simulink model "OnBoardMatlabExpo3"  (R2015b)
settings: Solver=FixedStepDiscrete  SolverMode=SingleTasking  StartTime=0.0  StopTime=10.0  FixedStep=0.002  RelTol=1e-3
PreLoadFcn:
  | waijung.modelPreload; % Required for working with Waijung Blockset. Do not remove.
undefined symbols (not defined in the file): CPHA_1Edge, CPOL_Low, Duplex, FirstBit_MSB, Full, Link, LQFP100, ST, STM32F407VG, STM32F4DISCOVERY
libraries: simulink x12, stm32f4_io_lib x7, cube_lib x3, stm32f4_spi_lib x3, stm32f4_device_config_lib x1, BC_USB x1, stm32f4_adc_lib x1
(part 1 of 2)
CloseFcn:
  | waijung.modelClose; % Required for working with Waijung Blockset. Do not remove.
settings Model: Creator=Hi  LastModifiedBy=Stefan
settings DataIOCC: SaveFormat=Array
settings OptimizationCC: OptimizeModelRefInitCode=on  LifeSpan=1
settings HardwareCC: ProdBitPerPointer=32  ProdLargestAtomicFloat=None  ProdIntDivRoundTo=Undefined  ProdWordSize=32  ProdHWDeviceType=ARM Compatible->Cortex - M4  TargetEndianess=LittleEndian  TargetHWDeviceType=ARM Compatible->Cortex - M4
settings RTWCC: SystemTargetFile=stm32f4.tlc  GenerateMakefile=off  TemplateMakefile=ert_default_tmf  Description=STM32F4 Target
settings CodeAppCC: ForceParamTrailComments=on  IgnoreCustomStorageClasses=off  OperatorAnnotations=on  SimulinkDataObjDesc=on  InsertBlockDesc=on  MATLABSourceComments=on
settings STFCustomTargetCC: ModelReferenceCompliant=off  ConcurrentExecutionCompliant=off  GeneratePreprocessorConditionals=Use local settings  CombineOutputUpdateFcns=on  ERTCustomFileBanners=on  SupportContinuousTime=off  SupportNonInlinedSFcns=off  MATLABClassNameForMDSCustomization=Simulink.SoftwareTarget.ERTCustomization  CPPClassGenCompliant=off  GRTInterface=off  SystemTargetFile=stm32f4.tlc
settings ERTTargetCC: ModelReferenceCompliant=off  ParMdlRefBuildCompliant=off  CompOptLevelCompliant=off  ConcurrentExecutionCompliant=off  ERTFirstTimeCompliant=off  ModelStepFunctionPrototypeControlCompliant=off  CPPClassGenCompliant=off  UseToolchainInfoCompliant=off  ERTSrcFileBannerTemplate=stm32f4_code_template.cgt  ERTHdrFileBannerTemplate=stm32f4_code_template.cgt  ERTDataSrcFileTemplate=stm32f4_code_template.cgt  ERTDataHdrFileTemplate=stm32f4_code_template.cgt  ERTCustomFileTemplate=stm32f4_file_process.tlc
settings ConfigComp: CovModelRefEnable=Off

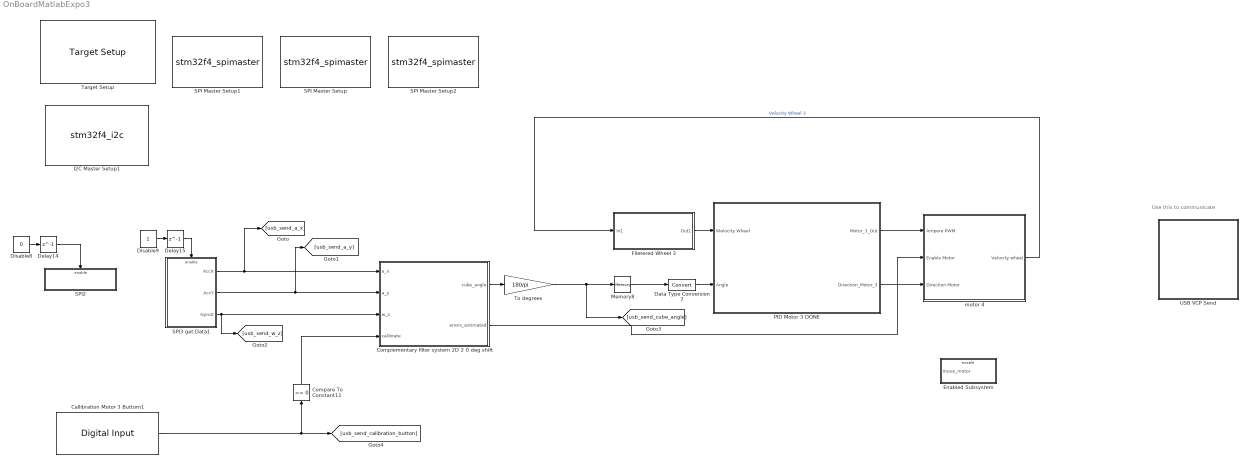
== system OnBoardMatlabExpo3 ==
  note: Use this to communicate
  Callibration Motor 3 Buttom1 : stm32f4_io_lib/Digital Input  port=E  speed=100  porttype=Pull Up  porttypestr=UP  use_pin0=off  use_pin1=off  use_pin2=off  use_pin3=off  use_pin4=off  use_pin5=off  use_pin6=off  use_pin7=off  use_pin8=off  use_pin9=off  use_pin10=on  use_pin11=off  use_pin12=off  use_pin13=off  use_pin14=off  use_pin15=off  pinstr=GPIO_Pin_10  usedpinarray="[0  0  0  0  0  0  0  0  0  0  1  0  0  0  0  0]"  bitbandingstr="#define CallibrationMotor3Buttom1_E10 Peripheral_BB(GPIOE->IDR, 10)  /* Output pin */"  sampletime=0.002  sampletimestr=0.002  blockid=CallibrationMotor3Buttom1  enablecustomportlabel=off  glabalinit=off  cinputportlabel=In1, In2  coutputportlabel=Out1, Out2
  Compare To Constant11 : simulink/Logic and Bit Operations/Compare To Constant  relop===  const=0  OutDataTypeStr=boolean  ZeroCross=off
  Complementary filter system 2D 2 0 deg shift : Subsystem  AncestorBlock=cube_lib/Complementary filter system 2D 2 0 deg shift
  Data Type Conversion7 : DataTypeConversion
  Delay14 : Delay  DelayLength=1  InitialCondition=1
  Delay15 : Delay  DelayLength=1  InitialCondition=0
  Disable8 : Constant  Value=0
  Disable9 : Constant
  Enabled Subsystem : Subsystem  TreatAsAtomicUnit=on
  Filetered Wheel 3 : Subsystem
  I2C Master Setup1 : S-Function  FunctionName=stm32f4_i2c  Parameters=configuration,module,transfer,clkspeed,timeout,sdapin,sclpin,writecount,readcount,inputtypearray,outputtypearray,confstr,sampletime,sampletimestr,blockid  SFunctionDeploymentMode=off  EnableBusSupport=off  mask(stm32f4_i2c){configuration=Setup, module=1, lastmodule=1, transfer=Blocking, dutycycle=TLow/THigh = 2, clkspeed=400, timeout=25, writecount=0, readcount=0, sdapin=B7, sclpin=B6, waitwritetime=0, inputtypearray=[0], outputtypearray=[0], confstr=["B","7","B","6","1","1","6","0","I2C_DutyCycle_2","0","off"], sampletime=-1, sampletimestr=0.002, blockid=I2CMasterSetup1}
      mask prompts: module "I2C Module"; lastmodule "Last module"; transfer "Transfer mode"; dutycycle "Duty cycle in fast mode"; clkspeed "Clock speed (kHz)"; timeout "Timeout (ms)"; writecount "Bytes write count"; readcount "Bytes read count"; sdapin "SDA pin"; sclpin "SCL pin"; waitwritetime "Wait write time (ms), default is 0"; inputtypearray "Input type array"; outputtypearray "Output type array"; confstr "Configuration string"; sampletime "Sample time (sec)"; sampletimestr "Compiled sample time (sec) in string"
      mask init:
      | stm32f4_i2c_callback('init');
      mask Help: web(fullfile(waijungdocroot,'stm32f4_i2c_setup.htm'), '-browser')
      mask TypeOptions configuration: Setup | Transaction
      mask Callback configuration: stm32f4_i2c_callback('configuration');
      mask TypeOptions module: 1 | 2 | 3
      mask Callback module: stm32f4_i2c_callback('module');
      mask TypeOptions transfer: Blocking | Non-blocking
      mask TypeOptions dutycycle: TLow/THigh = 16/9 | TLow/THigh = 2
      mask Callback dutycycle: stm32f4_i2c_callback('dutycycle');
      mask Callback writecount: stm32f4_i2c_callback('writecount');
      mask Callback readcount: stm32f4_i2c_callback('readcount');
      mask TypeOptions sdapin: - | B7 | B9
      mask Callback sdapin: stm32f4_i2c_callback('sdapin');
      mask TypeOptions sclpin: - | B6 | B8
      mask Callback sclpin: stm32f4_i2c_callback('sclpin');
      mask Callback confstr: stm32f4_i2c_callback('confstr');
      mask Callback sampletime: stm32f4_i2c_callback('sampletime');
      mask Callback sampletimestr: stm32f4_i2c_callback('sampletimestr');
      mask Callback blockid: stm32f4_i2c_callback('blockid');
      mask Display: text(0.5, 0.5, 'Module: I2C1\nClock: 400kHz\nSDA/SCL Pin: B7/B6','ver','middle','hor','center');
  Memory8 : Memory  InheritSampleTime=on
  "PID Motor 3 DONE " : Subsystem
  SPI Master Setup : S-Function  FunctionName=stm32f4_spimaster  Parameters=mode,configuration,module,datacount,inputtypearray,outputtypearray,confstr,sampletime,sampletimestr,blockid  SFunctionDeploymentMode=off  EnableBusSupport=off  mask(stm32f4_spimaster){configuration=Setup, module=2, mode=Write, lastmodule=2, direction=Full-Duplex, dataformat=8bit/ FirstBit_MSB, prescaler=32, lastpclk=42000000, baudrate=1312500, cpolcpha=CPOL_Low/ CPHA_1Edge, datacount=0, nssmode=Software, nsspin=Not used, softnssport=B, softnsspin=12, sckpin=B13, misopin=B14, mosipin=B15, pintype=Push Pull, pulltype=Pull Up, nssdelay=0, inputtypearray=[0], outputtypearray=[0], confstr=["SPI_Direction_2Lines_FullDuplex","8b","MSB","Low","1Edge","32","Soft","0","x","x","1","B","12","1","B","13","1","B","14","1","B","15","0","1","0","0","0","0","0","0","0","PP","0","UP"], sampletime=-1, sampletimestr=0.002, blockid=SPIMasterSetup}
      mask prompts: module "SPI Module:"; lastmodule "Last module:"; dataformat "Data format:"; prescaler "Buad rate prescaler: Pclk/"; lastpclk "Last PCLK"; baudrate "Baud rate (Hz)"; cpolcpha "Clock polarity (CPOL)/ Clock phase (CPHA):"; datacount "Data Write count:"; nssmode "Slave/chip select (nSS, nCS) mode"; nsspin "Slave/chip select (nSS, nCS) pin"; softnssport "Slave/chip select port (nSS, nCS)"; softnsspin "Slave/chip select pin (nSS, nCS)"; sckpin "SCLK pin:"; misopin "MISO pin:"; mosipin "MOSI pin:"; pintype "Pin type (Push-Pull/Open-Drain)"; pulltype "Pull Type (Up/Down)"; nssdelay "Data delay time, uS:"; inputtypearray "Input type array"; outputtypearray "Output type array"; confstr "Configuration string"; sampletime "Sample time (sec)"; sampletimestr "Compiled sample time (sec) in string"
      mask help:
      | Direction:
      |  - Full-Duplex, use this mode when need to send and receive data at same clock.
      |  - Half-Duplex_Tx, this mode is to transmit data to slave only. Pin MISO (Rx) can be free for other function.
      |  - Half-Duplex_Rx, this mode is to receive data from slave only. Pin MOSIO (Tx) can be free for other function.
      | Data format:
      |   This configuration is depending on the specification of slave device.
      | Baud rate prescaler:
      |  - Use this prescaler to devide from the PCLK for SPI clock.
      |  - This Prescaler value is auto determine corresponding to baudrate setting and selected SPI module.
      | Baud rate (Hz):
      |  - Select baud rate for SPI clock. Please check the maximum clock support for target slave device.
      | Clock polarity and Clock phase:
      |  - This configuration parameter is depending on slave device.
      |  - See waijung help for more description.
      | Slave/chip select mode:
      |  - Hardware, use hardware SPI module for slave select (or chip select) pin.
      |  - Software, this mode allow any available pin for slave select (or chip select) function.
      |  - Custom, SPI block did not control slave select pin. User may use Digital Output block to control by costom.
      mask init:
      | stm32f4_spimaster_callback('init');
      mask Help: web(fullfile(waijungdocroot,'stm32f4_spimaster_setup.htm'), '-browser')
      mask TypeOptions configuration: Setup | Transaction
      mask Callback configuration: stm32f4_spimaster_callback('configuration');
      mask TypeOptions module: 1 | 2 | 3
      mask Callback module: stm32f4_spimaster_callback('module');
      mask TypeOptions mode: Read/ Write | Read | Write
      mask Callback mode: stm32f4_spimaster_callback('mode');
      mask TypeOptions direction: Full-Duplex | Half-Duplex_Tx | Half-Duplex_Rx
      mask Callback direction: stm32f4_spimaster_callback('direction');
      mask TypeOptions dataformat: 8bit/ FirstBit_MSB | 8bit/ FirstBit_LSB | 16bit/ FirstBit_MSB | 16bit/ FirstBit_LSB
      mask TypeOptions prescaler: 2 | 4 | 8 | 16 | 32 | 64 | 128 | 256
      mask TypeOptions baudrate: Not set | 21000000 | 10500000 | 5250000 | 2625000 | 1312500 | 656250 | 328125 | 164063
      mask Callback baudrate: stm32f4_spimaster_callback('baudrate');
      mask TypeOptions cpolcpha: CPOL_Low/ CPHA_1Edge | CPOL_Low/ CPHA_2Edge | CPOL_High/ CPHA_1Edge | CPOL_High/ CPHA_2Edge
      mask Callback datacount: stm32f4_spimaster_callback('datacount');
      mask TypeOptions nssmode: Hardware | Software | Custom
      mask Callback nssmode: stm32f4_spimaster_callback('nssmode');
      mask TypeOptions nsspin: Not used | B9 | B12
      mask TypeOptions softnssport: A | B | C | D | E | F | G | H | I
      mask TypeOptions softnsspin: 0 | 1 | 2 | 3 | 4 | 5 | 6 | 7 | 8 | 9 | 10 | 11 | 12 | 13 | 14 | 15
      mask TypeOptions sckpin: Not used | B10 | B13
      mask TypeOptions misopin: Not used | B14 | C2
      mask TypeOptions mosipin: Not used | B15 | C3
      mask TypeOptions pintype: Push Pull | Open Drain
      mask TypeOptions pulltype: None | Pull Up | Pull Down
      mask Callback confstr: stm32f4_spimaster_callback('confstr');
      mask Callback sampletime: stm32f4_spimaster_callback('sampletime');
      mask Callback sampletimestr: stm32f4_spimaster_callback('sampletimestr');
      mask Callback blockid: stm32f4_spimaster_callback('blockid');
      mask Display: text(0.5, 0.5, 'Module: SPI2 (Master)\nFull-Duplex\nBaudrate: 1312500','ver','middle','hor','center');
  SPI Master Setup1 : S-Function  FunctionName=stm32f4_spimaster  Parameters=mode,configuration,module,datacount,inputtypearray,outputtypearray,confstr,sampletime,sampletimestr,blockid  SFunctionDeploymentMode=off  EnableBusSupport=off  mask(stm32f4_spimaster){configuration=Setup, module=1, mode=Write, lastmodule=1, direction=Full-Duplex, dataformat=8bit/ FirstBit_MSB, prescaler=64, lastpclk=84000000, baudrate=1312500, cpolcpha=CPOL_Low/ CPHA_1Edge, datacount=0, nssmode=Software, nsspin=Not used, softnssport=C, softnsspin=5, sckpin=A5, misopin=A6, mosipin=A7, pintype=Push Pull, pulltype=Pull Up, nssdelay=0, inputtypearray=[0], outputtypearray=[0], confstr=["SPI_Direction_2Lines_FullDuplex","8b","MSB","Low","1Edge","64","Soft","0","x","x","1","C","5","1","A","5","1","A","6","1","A","7","1","0","1","0","0","0","0","0","0","PP","0","UP"], sampletime=-1, sampletimestr=0.002, blockid=SPIMasterSetup1}
      mask prompts: module "SPI Module:"; lastmodule "Last module:"; dataformat "Data format:"; prescaler "Buad rate prescaler: Pclk/"; lastpclk "Last PCLK"; baudrate "Baud rate (Hz)"; cpolcpha "Clock polarity (CPOL)/ Clock phase (CPHA):"; datacount "Data Write count:"; nssmode "Slave/chip select (nSS, nCS) mode"; nsspin "Slave/chip select (nSS, nCS) pin"; softnssport "Slave/chip select port (nSS, nCS)"; softnsspin "Slave/chip select pin (nSS, nCS)"; sckpin "SCLK pin:"; misopin "MISO pin:"; mosipin "MOSI pin:"; pintype "Pin type (Push-Pull/Open-Drain)"; pulltype "Pull Type (Up/Down)"; nssdelay "Data delay time, uS:"; inputtypearray "Input type array"; outputtypearray "Output type array"; confstr "Configuration string"; sampletime "Sample time (sec)"; sampletimestr "Compiled sample time (sec) in string"
      mask help:
      | Direction:
      |  - Full-Duplex, use this mode when need to send and receive data at same clock.
      |  - Half-Duplex_Tx, this mode is to transmit data to slave only. Pin MISO (Rx) can be free for other function.
      |  - Half-Duplex_Rx, this mode is to receive data from slave only. Pin MOSIO (Tx) can be free for other function.
      | Data format:
      |   This configuration is depending on the specification of slave device.
      | Baud rate prescaler:
      |  - Use this prescaler to devide from the PCLK for SPI clock.
      |  - This Prescaler value is auto determine corresponding to baudrate setting and selected SPI module.
      | Baud rate (Hz):
      |  - Select baud rate for SPI clock. Please check the maximum clock support for target slave device.
      | Clock polarity and Clock phase:
      |  - This configuration parameter is depending on slave device.
      |  - See waijung help for more description.
      | Slave/chip select mode:
      |  - Hardware, use hardware SPI module for slave select (or chip select) pin.
      |  - Software, this mode allow any available pin for slave select (or chip select) function.
      |  - Custom, SPI block did not control slave select pin. User may use Digital Output block to control by costom.
      mask init:
      | stm32f4_spimaster_callback('init');
      mask Help: web(fullfile(waijungdocroot,'stm32f4_spimaster_setup.htm'), '-browser')
      mask TypeOptions configuration: Setup | Transaction
      mask Callback configuration: stm32f4_spimaster_callback('configuration');
      mask TypeOptions module: 1 | 2 | 3
      mask Callback module: stm32f4_spimaster_callback('module');
      mask TypeOptions mode: Read/ Write | Read | Write
      mask Callback mode: stm32f4_spimaster_callback('mode');
      mask TypeOptions direction: Full-Duplex | Half-Duplex_Tx | Half-Duplex_Rx
      mask Callback direction: stm32f4_spimaster_callback('direction');
      mask TypeOptions dataformat: 8bit/ FirstBit_MSB | 8bit/ FirstBit_LSB | 16bit/ FirstBit_MSB | 16bit/ FirstBit_LSB
      mask TypeOptions prescaler: 2 | 4 | 8 | 16 | 32 | 64 | 128 | 256
      mask TypeOptions baudrate: Not set | 42000000 | 21000000 | 10500000 | 5250000 | 2625000 | 1312500 | 656250 | 328125
      mask Callback baudrate: stm32f4_spimaster_callback('baudrate');
      mask TypeOptions cpolcpha: CPOL_Low/ CPHA_1Edge | CPOL_Low/ CPHA_2Edge | CPOL_High/ CPHA_1Edge | CPOL_High/ CPHA_2Edge
      mask Callback datacount: stm32f4_spimaster_callback('datacount');
      mask TypeOptions nssmode: Hardware | Software | Custom
      mask Callback nssmode: stm32f4_spimaster_callback('nssmode');
      mask TypeOptions nsspin: Not used | A4 | A15
      mask TypeOptions softnssport: A | B | C | D | E | F | G | H | I
      mask TypeOptions softnsspin: 0 | 1 | 2 | 3 | 4 | 5 | 6 | 7 | 8 | 9 | 10 | 11 | 12 | 13 | 14 | 15
      mask TypeOptions sckpin: Not used | A5 | B3
      mask TypeOptions misopin: Not used | A6 | B4
      mask TypeOptions mosipin: Not used | A7 | B5
      mask TypeOptions pintype: Push Pull | Open Drain
      mask TypeOptions pulltype: None | Pull Up | Pull Down
      mask Callback confstr: stm32f4_spimaster_callback('confstr');
      mask Callback sampletime: stm32f4_spimaster_callback('sampletime');
      mask Callback sampletimestr: stm32f4_spimaster_callback('sampletimestr');
      mask Callback blockid: stm32f4_spimaster_callback('blockid');
      mask Display: text(0.5, 0.5, 'Module: SPI1 (Master)\nFull-Duplex\nBaudrate: 1312500','ver','middle','hor','center');
  SPI Master Setup2 : S-Function  FunctionName=stm32f4_spimaster  Parameters=mode,configuration,module,datacount,inputtypearray,outputtypearray,confstr,sampletime,sampletimestr,blockid  SFunctionDeploymentMode=off  EnableBusSupport=off  mask(stm32f4_spimaster){configuration=Setup, module=3, mode=Write, lastmodule=3, direction=Full-Duplex, dataformat=8bit/ FirstBit_MSB, prescaler=32, lastpclk=42000000, baudrate=1312500, cpolcpha=CPOL_Low/ CPHA_1Edge, datacount=0, nssmode=Software, nsspin=Not used, softnssport=C, softnsspin=11, sckpin=C10, misopin=B4, mosipin=B5, pintype=Push Pull, pulltype=Pull Up, nssdelay=0, inputtypearray=[0], outputtypearray=[0], confstr=["SPI_Direction_2Lines_FullDuplex","8b","MSB","Low","1Edge","32","Soft","0","x","x","1","C","11","1","C","10","1","B","4","1","B","5","0","1","1","0","0","0","0","0","0","PP","0","UP"], sampletime=-1, sampletimestr=0.002, blockid=SPIMasterSetup2}
      mask prompts: module "SPI Module:"; lastmodule "Last module:"; dataformat "Data format:"; prescaler "Buad rate prescaler: Pclk/"; lastpclk "Last PCLK"; baudrate "Baud rate (Hz)"; cpolcpha "Clock polarity (CPOL)/ Clock phase (CPHA):"; datacount "Data Write count:"; nssmode "Slave/chip select (nSS, nCS) mode"; nsspin "Slave/chip select (nSS, nCS) pin"; softnssport "Slave/chip select port (nSS, nCS)"; softnsspin "Slave/chip select pin (nSS, nCS)"; sckpin "SCLK pin:"; misopin "MISO pin:"; mosipin "MOSI pin:"; pintype "Pin type (Push-Pull/Open-Drain)"; pulltype "Pull Type (Up/Down)"; nssdelay "Data delay time, uS:"; inputtypearray "Input type array"; outputtypearray "Output type array"; confstr "Configuration string"; sampletime "Sample time (sec)"; sampletimestr "Compiled sample time (sec) in string"
      mask help:
      | Direction:
      |  - Full-Duplex, use this mode when need to send and receive data at same clock.
      |  - Half-Duplex_Tx, this mode is to transmit data to slave only. Pin MISO (Rx) can be free for other function.
      |  - Half-Duplex_Rx, this mode is to receive data from slave only. Pin MOSIO (Tx) can be free for other function.
      | Data format:
      |   This configuration is depending on the specification of slave device.
      | Baud rate prescaler:
      |  - Use this prescaler to devide from the PCLK for SPI clock.
      |  - This Prescaler value is auto determine corresponding to baudrate setting and selected SPI module.
      | Baud rate (Hz):
      |  - Select baud rate for SPI clock. Please check the maximum clock support for target slave device.
      | Clock polarity and Clock phase:
      |  - This configuration parameter is depending on slave device.
      |  - See waijung help for more description.
      | Slave/chip select mode:
      |  - Hardware, use hardware SPI module for slave select (or chip select) pin.
      |  - Software, this mode allow any available pin for slave select (or chip select) function.
      |  - Custom, SPI block did not control slave select pin. User may use Digital Output block to control by costom.
      mask init:
      | stm32f4_spimaster_callback('init');
      mask Help: web(fullfile(waijungdocroot,'stm32f4_spimaster_setup.htm'), '-browser')
      mask TypeOptions configuration: Setup | Transaction
      mask Callback configuration: stm32f4_spimaster_callback('configuration');
      mask TypeOptions module: 1 | 2 | 3
      mask Callback module: stm32f4_spimaster_callback('module');
      mask TypeOptions mode: Read/ Write | Read | Write
      mask Callback mode: stm32f4_spimaster_callback('mode');
      mask TypeOptions direction: Full-Duplex | Half-Duplex_Tx | Half-Duplex_Rx
      mask Callback direction: stm32f4_spimaster_callback('direction');
      mask TypeOptions dataformat: 8bit/ FirstBit_MSB | 8bit/ FirstBit_LSB | 16bit/ FirstBit_MSB | 16bit/ FirstBit_LSB
      mask TypeOptions prescaler: 2 | 4 | 8 | 16 | 32 | 64 | 128 | 256
      mask TypeOptions baudrate: Not set | 21000000 | 10500000 | 5250000 | 2625000 | 1312500 | 656250 | 328125 | 164063
      mask Callback baudrate: stm32f4_spimaster_callback('baudrate');
      mask TypeOptions cpolcpha: CPOL_Low/ CPHA_1Edge | CPOL_Low/ CPHA_2Edge | CPOL_High/ CPHA_1Edge | CPOL_High/ CPHA_2Edge
      mask Callback datacount: stm32f4_spimaster_callback('datacount');
      mask TypeOptions nssmode: Hardware | Software | Custom
      mask Callback nssmode: stm32f4_spimaster_callback('nssmode');
      mask TypeOptions nsspin: Not used | A4 | A15
      mask TypeOptions softnssport: A | B | C | D | E | F | G | H | I
      mask TypeOptions softnsspin: 0 | 1 | 2 | 3 | 4 | 5 | 6 | 7 | 8 | 9 | 10 | 11 | 12 | 13 | 14 | 15
      mask TypeOptions sckpin: Not used | B3 | C10
      mask TypeOptions misopin: Not used | B4 | C11
      mask TypeOptions mosipin: Not used | B5 | C12
      mask TypeOptions pintype: Push Pull | Open Drain
      mask TypeOptions pulltype: None | Pull Up | Pull Down
      mask Callback confstr: stm32f4_spimaster_callback('confstr');
      mask Callback sampletime: stm32f4_spimaster_callback('sampletime');
      mask Callback sampletimestr: stm32f4_spimaster_callback('sampletimestr');
      mask Callback blockid: stm32f4_spimaster_callback('blockid');
      mask Display: text(0.5, 0.5, 'Module: SPI3 (Master)\nFull-Duplex\nBaudrate: 1312500','ver','middle','hor','center');
  SPI2 : Subsystem  Priority=0  TreatAsAtomicUnit=on
  SPI3 get Data1 : Subsystem
  Target Setup : stm32f4_device_config_lib/Target Setup  Priority=100  compiler=GNU ARM  previous_compiler=GNU ARM  mcu=STM32F407VG (LQFP100); STM32F4DISCOVERY  mcustr=STM32F407VG  clockconfig=STM32F4DISCOVERY Default (HSEOSC-8MHz/HCLK-168MHz)  system_stm32f4xx_c_path=C:\Users\Jasper Gundersen\Documents\Cube\waijung15_04a\targets\stm32f4_target\stm32f4\utils\STM32F4xx_AN3988_V1.0.1\stm32f4_default\hseosc8mhz  showmemoryconfiguration=off  stacksize=0x400  heapsize=0x200  enableautocompiledownload=on  fullchiperase=off  programmerinterface=ST-Link  editctrlstr=on  compilercontrolstr=$(patsubst %, -I%, .) -mcpu=cortex-m4 -mthumb -mthumb-interwork -mfloat-abi=hard -mfpu=fpv4-sp-d16 -ffast-math -Wall -Wextra -Ofast  assemblercontrolstr=$(patsubst %, -I%, .) -mcpu=cortex-m4 -mthumb -mthumb-interwork -mfloat-abi=hard -mfpu=fpv4-sp-d16 -ffast-math -Wall -Wextra -Ofast -Wa,-amhls=$(<:.s=.lst) -D__STACK_SIZE=$(STACK_SIZE) -D__HEAP_SIZE=$(HEAP_SIZE)  linkercontrolstr=-T$(LD_SCRIPT) -g -Wl,-Map=$(MAP),--cref,--no-warn-mismatch -mcpu=cortex-m4 -mthumb -mthumb-interwork -mfloat-abi=hard -mfpu=fpv4-sp-d16  runafterdownload=on  execprofile=None  profileruart=1  profilerbaud=115200  profilertxpin=Not used  profilerinitstr=0.002,168000000,336000,115200,0  manualsetsampletime=on  sampletime=0.002  blockid=TargetSetup  systickreloadvalue=336000  hseval=8000000  lastprofileruart=1  hclk=168000000  flashorigin=0x8000000  flashlength=1M  ramorigin=0x20000000  ramlength=112k  useextram=off
  To degrees : Gain  Gain=180/pi
  USB VCP Send : Subsystem
  motor 4 : Subsystem
  wires:
  Delay14/1 -> SPI2/Enable
  Disable8/1 -> Delay14/1
  Disable9/1 -> Delay15/1
  Delay15/1 -> SPI3 get Data1/Enable
  Callibration Motor 3 Buttom1/1 -> [usb_send_calibration_button], Compare To Constant11/1
  SPI3 get Data1/3(GyroZ) -> Complementary filter system 2D 2 0 deg shift/3(w_z), [usb_send_w_z]
  motor 4/1(Velocity wheel) -> Filetered Wheel 3/1(In1)  "Velocity Wheel 3"
  Filetered Wheel 3/1(Out1) -> "PID Motor 3 DONE "/1("Welocity Wheel ")
  Data Type Conversion7/1 -> "PID Motor 3 DONE "/2(Angle)
  "PID Motor 3 DONE "/1(Motor_3_Out) -> motor 4/1(Ampere PWM)
  Memory8/1 -> Data Type Conversion7/1
  "PID Motor 3 DONE "/2("Direction_Motor_3 ") -> motor 4/3("Direction Motor ")
  Compare To Constant11/1 -> Complementary filter system 2D 2 0 deg shift/4(calibrate)
  SPI3 get Data1/1(AccX) -> Complementary filter system 2D 2 0 deg shift/1(a_x), [usb_send_a_x]
  SPI3 get Data1/2("AccY ") -> Complementary filter system 2D 2 0 deg shift/2(a_y), [usb_send_a_y]
  Complementary filter system 2D 2 0 deg shift/1(cube_angle) -> To degrees/1
  Complementary filter system 2D 2 0 deg shift/2(errors_estimated) -> motor 4/2(Enable Motor)
  To degrees/1 -> [usb_send_cube_angle], Memory8/1

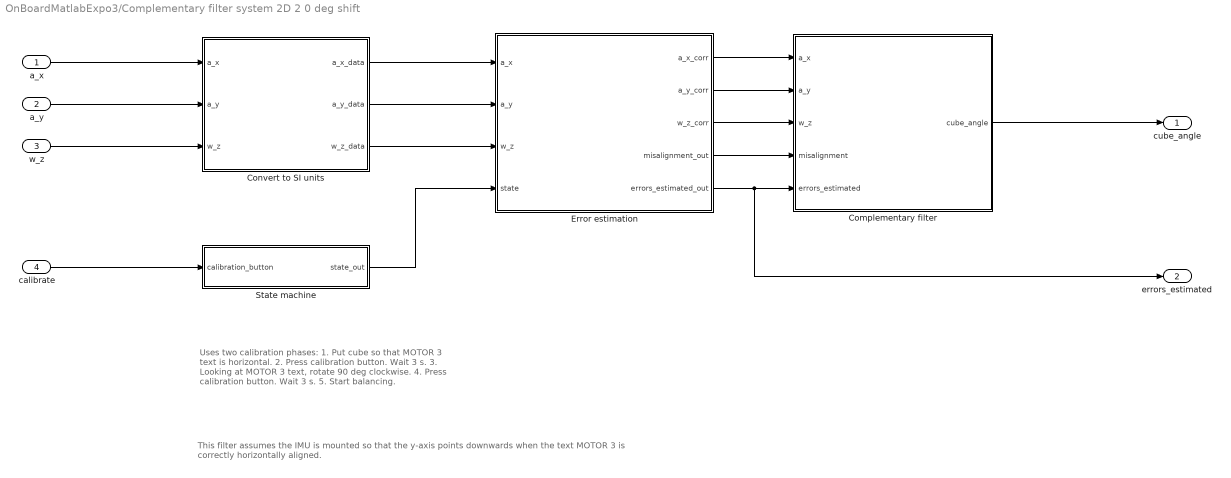
== system OnBoardMatlabExpo3/Complementary filter system 2D 2 0 deg shift ==
  note: Uses two calibration phases:
      | 1. Put cube so that MOTOR 3 text is horizontal.
      | 2. Press calibration button. Wait 3 s.
      | 3. Looking at MOTOR 3 text, rotate 90 deg clockwise.
      | 4. Press calibration button. Wait 3 s.
      | 5. Start balancing.
  note: This filter assumes the IMU is mounted so that the y-axis points downwards when the text MOTOR 3 is correctly horizontally aligned.
  a_x : Inport
  a_y : Inport  Port=2
  w_z : Inport  Port=3
  calibrate : Inport  Port=4
  Complementary filter : MATLAB Function  TreatAsAtomicUnit=on
  Convert to SI units : MATLAB Function  TreatAsAtomicUnit=on
  Error estimation : MATLAB Function  TreatAsAtomicUnit=on
  State machine : MATLAB Function  TreatAsAtomicUnit=on
  cube_angle : Outport
  errors_estimated : Outport  Port=2
  wires:
  State machine/1(state_out) -> Error estimation/4(state)
  calibrate/1 -> State machine/1(calibration_button)
  Error estimation/4(misalignment_out) -> Complementary filter/4(misalignment)
  Error estimation/3(w_z_corr) -> Complementary filter/3(w_z)
  Error estimation/2(a_y_corr) -> Complementary filter/2(a_y)
  Error estimation/5(errors_estimated_out) -> errors_estimated/1, Complementary filter/5(errors_estimated)
  Error estimation/1(a_x_corr) -> Complementary filter/1(a_x)
  Convert to SI units/3(w_z_data) -> Error estimation/3(w_z)
  Convert to SI units/2(a_y_data) -> Error estimation/2(a_y)
  Convert to SI units/1(a_x_data) -> Error estimation/1(a_x)
  a_y/1 -> Convert to SI units/2(a_y)
  a_x/1 -> Convert to SI units/1(a_x)
  w_z/1 -> Convert to SI units/3(w_z)
  Complementary filter/1(cube_angle) -> cube_angle/1

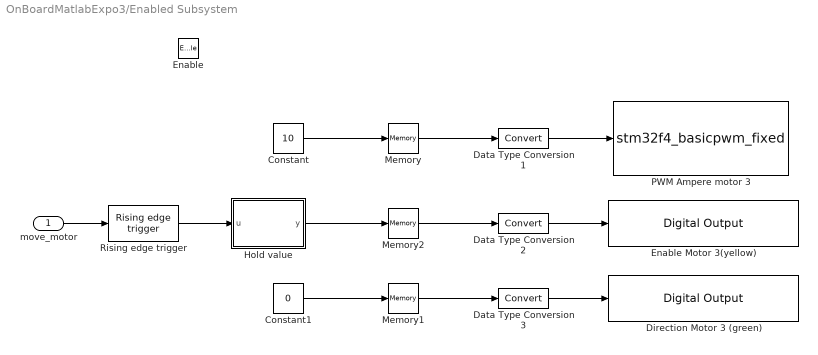
== system OnBoardMatlabExpo3/Enabled Subsystem ==
  move_motor : Inport
  Enable : EnablePort
  Constant : Constant  Value=10
  Constant1 : Constant  Value=0
  Data Type Conversion1 : DataTypeConversion
  Data Type Conversion2 : DataTypeConversion
  Data Type Conversion3 : DataTypeConversion
  Direction Motor 3 (green) : stm32f4_io_lib/Digital Output  use_bitband=on  port=D  speed=100  porttype=Push Pull  porttypestr=PP  use_pin0=off  use_pin1=off  use_pin2=off  use_pin3=off  use_pin4=off  use_pin5=off  use_pin6=off  use_pin7=off  use_pin8=off  use_pin9=off  use_pin10=off  use_pin11=on  use_pin12=off  use_pin13=off  use_pin14=off  use_pin15=off  pinstr=GPIO_Pin_11  usedpinarray="[0  0  0  0  0  0  0  0  0  0  0  1  0  0  0  0]"  bitbandingstr="#define motor4DirectionMotor3green_D11 Peripheral_BB(GPIOD->ODR, 11)  /* Output pin */"  sampletime=-1  sampletimestr=0.002  blockid=motor4DirectionMotor3green  enablecustomportlabel=off  globalinit=off  cinputportlabel=In1, In2  coutputportlabel=0
  Enable Motor 3(yellow) : stm32f4_io_lib/Digital Output  use_bitband=on  port=D  speed=100  porttype=Push Pull  porttypestr=PP  use_pin0=off  use_pin1=off  use_pin2=off  use_pin3=off  use_pin4=off  use_pin5=off  use_pin6=off  use_pin7=off  use_pin8=off  use_pin9=on  use_pin10=off  use_pin11=off  use_pin12=off  use_pin13=off  use_pin14=off  use_pin15=off  pinstr=GPIO_Pin_9  usedpinarray="[0  0  0  0  0  0  0  0  0  1  0  0  0  0  0  0]"  bitbandingstr="#define motor4EnableMotor3yellow_D9 Peripheral_BB(GPIOD->ODR, 9)  /* Output pin */"  sampletime=-1  sampletimestr=0.002  blockid=motor4EnableMotor3yellow  enablecustomportlabel=off  globalinit=off  cinputportlabel=In1, In2  coutputportlabel=0
  Hold value : MATLAB Function  TreatAsAtomicUnit=on
  Memory : Memory  InheritSampleTime=on
  Memory1 : Memory  InheritSampleTime=on
  Memory2 : Memory  InheritSampleTime=on
  PWM Ampere motor 3 : S-Function  FunctionName=stm32f4_basicpwm_fixed  Parameters=timer,pwmperiod,uc3m_pwmperiod,ch1pin,ch2pin,ch3pin,ch4pin,sampletime,sampletimestr,blockid,apb,portstr,pinstr,pinmat,timarr,timprescale,chmat,polaritystr  SFunctionDeploymentMode=off  EnableBusSupport=off  mask(stm32f4_basicpwm_fixed){timer=2, pwmperiod=0.02, uc3m_pwmperiod=0.0002, polarity=Active High, polaritystr=TIM_OCPolarity_High, ch1pin=Not available - Do not use, ch2pin=Not available - Do not use, ch3pin=Not available - Do not use, ch4pin=A3, sampletime=0.002, sampletimestr=0.002, blockid=motor4PWMAmperemotor3, portpinstr=,,,A3, enablecustomportlabel=off, cinputportlabel=In1, In2, In3, In4, coutputportlabel=0, callbackgensrccode=off, apb=1, portstr=["A"], pinstr=["GPIO_Pin_3"], pinmat=[1 3], timarr=59999, timprescale=55, chmat=[4]}
      mask prompts: pwmperiod "PWM Period (seconds)"; uc3m_pwmperiod "PWM Signal Period (seconds)"; ch1pin "Channel 1"; ch2pin "Channel 2"; ch3pin "Channel 3"; ch4pin "Channel 4"; sampletime "Sample time (sec)"; sampletimestr "Compiled sample time (sec) in string"; portpinstr "Port pin string"; enablecustomportlabel "Enable custom port labels"; cinputportlabel "Custom input port labels (Ex. In1, In2, In3)"; coutputportlabel "Custom output port labels (Ex. Out1, Out2, Out3)"; callbackgensrccode "Gen source code from callback"; portstr "Port string"; pinstr "Pin string"; pinmat "Pin matrix"; timarr "Timer ARR"; timprescale "Timer PRESCALE"; chmat "Channel order"
      mask help:
      | This block implements basic Edge-aligned Pulse Width Modulation (PWM) generation.
      | All timers are 16-bit. The PWM period is fixed (per timer).
      |
      | This block was fixed by Sr Antonio
      mask init:
      | stm32f4_basicpwm_callback_fixed('init');
      mask Help: web(fullfile(waijungdocroot,'stm32f4_basicpwm.htm'),'-browser')
      mask TypeOptions timer: 1 | 2 | 3 | 4 | 5 | 8 | 9 | 10 | 11 | 12 | 13 | 14
      mask Callback timer: stm32f4_basicpwm_callback_fixed('timer');
      mask Callback pwmperiod: stm32f4_basicpwm_callback_fixed('pwmperiod');
      mask Callback uc3m_pwmperiod: stm32f4_basicpwm_callback_fixed('uc3m_pwmperiod');
      mask TypeOptions polarity: Active High | Active Low
      mask Callback polarity: stm32f4_basicpwm_callback_fixed('polarity');
      mask TypeOptions ch1pin: Not available - Do not use | A0 | A5
      mask Callback ch1pin: stm32f4_basicpwm_callback_fixed('ch1pin');
      mask TypeOptions ch2pin: Not available - Do not use | A1 | B3
      mask Callback ch2pin: stm32f4_basicpwm_callback_fixed('ch2pin');
      mask TypeOptions ch3pin: Not available - Do not use | A2 | B10
      mask Callback ch3pin: stm32f4_basicpwm_callback_fixed('ch3pin');
      mask TypeOptions ch4pin: Not available - Do not use | A3 | B11
      mask Callback ch4pin: stm32f4_basicpwm_callback_fixed('ch4pin');
      mask Callback sampletime: stm32f4_basicpwm_callback_fixed('sampletime');
      mask Callback sampletimestr: stm32f4_basicpwm_callback_fixed('sampletimestr');
      mask Callback blockid: stm32f4_basicpwm_callback_fixed('blockid');
      mask Callback enablecustomportlabel: stm32f4_basicpwm_callback_fixed('enablecustomportlabel')
      mask Display: text(0.95, 0.5, 'UC3M FIXED\nTimer: 2\nPolarity: Active High\nPeriod (sec): 0.0002\nTs (sec): 0.002','ver','middle','hor','right');port_label('input', 1,'CH4 (A3)')
  Rising edge trigger : cube_lib/Rising edge trigger
  wires:
  Constant/1 -> Memory/1
  Data Type Conversion3/1 -> Direction Motor 3 (green)/1
  Data Type Conversion2/1 -> Enable Motor 3(yellow)/1
  Memory/1 -> Data Type Conversion1/1
  Memory2/1 -> Data Type Conversion2/1
  Constant1/1 -> Memory1/1
  Memory1/1 -> Data Type Conversion3/1
  Rising edge trigger/1 -> Hold value/1(u)
  Data Type Conversion1/1 -> PWM Ampere motor 3/1
  move_motor/1 -> Rising edge trigger/1
  Hold value/1(y) -> Memory2/1

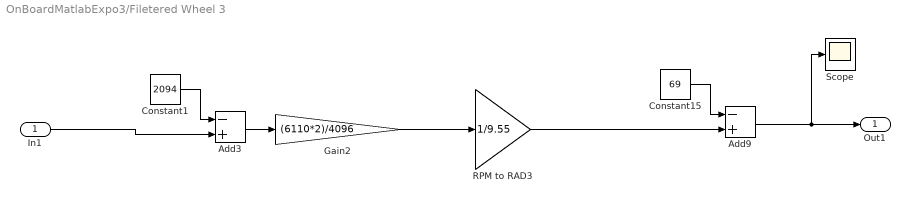
== system OnBoardMatlabExpo3/Filetered Wheel 3 ==
  In1 : Inport
  Add3 : Sum  Inputs=-+
  Add9 : Sum  Inputs=-+
  Constant1 : Constant  Value=2094  SampleTime=-1
  Constant15 : Constant  Value=69  SampleTime=-1
  Gain2 : Gain  Gain=(6110*2)/4096
  RPM to RAD3 : Gain  Gain=1/9.55
  Scope : Scope
  Out1 : Outport
  wires:
  Gain2/1 -> RPM to RAD3/1
  Add3/1 -> Gain2/1
  Constant1/1 -> Add3/1
  In1/1 -> Add3/2
  Constant15/1 -> Add9/1
  RPM to RAD3/1 -> Add9/2
  Add9/1 -> Scope/1, Out1/1

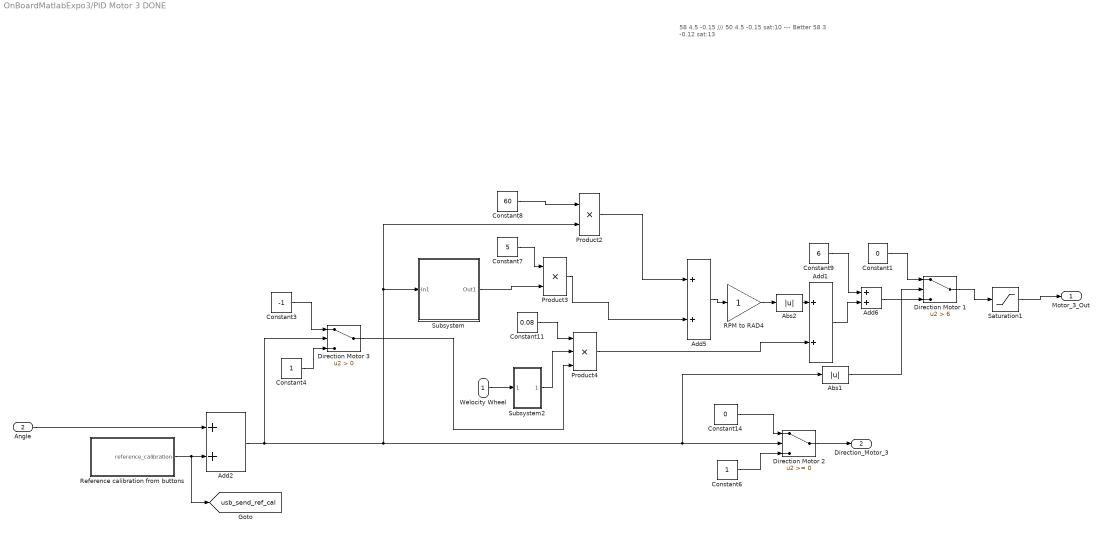
== system OnBoardMatlabExpo3/PID Motor 3 DONE  ==
  note: 58
      | 4.5
      | -0.15
      | ///
      | 50
      | 4.5
      | -0.15
      | sat:10
      | --- Better
      | 58
      | 3
      | -0.12
      | sat:13
  "Welocity Wheel " : Inport
  Angle : Inport  Port=2
  Abs1 : Abs
  Abs2 : Abs
  Add{1..2,5..6} (4 alike) : Sum
  Constant1 : Constant  Value=0  OutDataTypeStr=single  SampleTime=-1
  Constant11 : Constant  Value=0.08  OutDataTypeStr=single  SampleTime=-1
  Constant14 : Constant  Value=0  OutDataTypeStr=single  SampleTime=-1
  Constant3 : Constant  Value=-1  OutDataTypeStr=single  SampleTime=-1
  Constant4 : Constant  OutDataTypeStr=single  SampleTime=-1
  Constant6 : Constant  OutDataTypeStr=single  SampleTime=-1
  Constant7 : Constant  Value=5  OutDataTypeStr=single  SampleTime=-1
  Constant8 : Constant  Value=60  OutDataTypeStr=single  SampleTime=-1
  Constant9 : Constant  Value=6  SampleTime=-1
  Direction Motor 1 : Switch  Criteria=u2 > Threshold  Threshold=6
  Direction Motor 2 : Switch
  Direction Motor 3 : Switch  Criteria=u2 > Threshold
  Product2 : Product
  Product3 : Product
  Product4 : Product  Inputs=3
  RPM to RAD4 : Gain
  Reference calibration from buttons : Subsystem
  Saturation1 : Saturate  UpperLimit=90  LowerLimit=10
  Subsystem : Subsystem
  Subsystem2 : Subsystem
  Motor_3_Out : Outport
  "Direction_Motor_3 " : Outport  Port=2
  tag scope: usb_send_ref_cal=global
  wires:
  Direction Motor 2/1 -> "Direction_Motor_3 "/1
  Constant7/1 -> Product3/1
  Constant11/1 -> Product4/1
  Constant14/1 -> Direction Motor 2/1
  Constant6/1 -> Direction Motor 2/3
  Product3/1 -> Add5/2
  Constant9/1 -> Add6/1
  Add5/1 -> RPM to RAD4/1
  RPM to RAD4/1 -> Abs2/1
  Product2/1 -> Add5/1
  Abs2/1 -> Add1/1
  Saturation1/1 -> Motor_3_Out/1
  Constant8/1 -> Product2/1
  Add6/1 -> Direction Motor 1/3
  Direction Motor 1/1 -> Saturation1/1
  Constant1/1 -> Direction Motor 1/1
  Abs1/1 -> Direction Motor 1/2
  Product4/1 -> Add1/2
  "Welocity Wheel "/1 -> Subsystem2/1(In1)
  Angle/1 -> Add2/1
  Subsystem/1(Out1) -> Product3/2
  Add1/1 -> Add6/2
  Constant4/1 -> Direction Motor 3/3
  Constant3/1 -> Direction Motor 3/1
  Direction Motor 3/1 -> Product4/3
  Subsystem2/1(Out2) -> Product4/2
  Add2/1 -> Direction Motor 3/2, Subsystem/1(In1), Product2/2, Abs1/1, Direction Motor 2/2
  Reference calibration from buttons/1(reference_calibration) -> [usb_send_ref_cal], Add2/2

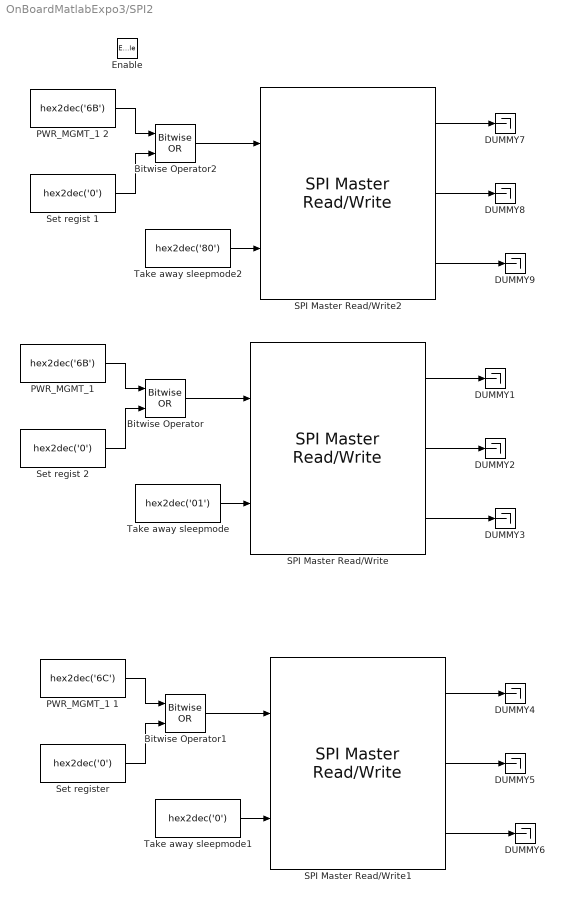
== system OnBoardMatlabExpo3/SPI2 ==
  Enable : EnablePort
  Bitwise Operator : simulink/Logic and Bit Operations/Bitwise Operator  logicop=OR  UseBitMask=off  NumInputPorts=2  BitMask=bin2dec('11011001')  BitMaskRealWorld=Stored Integer
  Bitwise Operator1 : simulink/Logic and Bit Operations/Bitwise Operator  logicop=OR  UseBitMask=off  NumInputPorts=2  BitMask=bin2dec('11011001')  BitMaskRealWorld=Stored Integer
  Bitwise Operator2 : simulink/Logic and Bit Operations/Bitwise Operator  logicop=OR  UseBitMask=off  NumInputPorts=2  BitMask=bin2dec('11011001')  BitMaskRealWorld=Stored Integer
  DUMMY{1..9} (9 alike) : Terminator
  "PWR_MGMT_1 " : Constant  Value=hex2dec('6B')  OutDataTypeStr=uint8
  PWR_MGMT_1 1 : Constant  Value=hex2dec('6C')  OutDataTypeStr=uint8
  PWR_MGMT_1 2 : Constant  Value=hex2dec('6B')  OutDataTypeStr=uint8
  SPI Master Read/Write : stm32f4_spi_lib/SPI Master Read//Write  configuration=Transaction  module=3  mode=Read/ Write  lastmodule=1  direction=Full-Duplex  dataformat=8bit/ FirstBit_MSB  prescaler=4  cpolcpha=CPOL_Low/ CPHA_1Edge  datacount=2  nssmode=Custom  nsspin=Not used  softnssport=E  softnsspin=0  sckpin=A5  misopin=A6  mosipin=A7  inputtypearray=[2 3 3]  outputtypearray=[3 7 3 3]  confstr="[\"SPI_Direction_2Lines_FullDuplex\",\"8b\",\"MSB\",\"Low\",\"1Edge\",\"4\",\"Soft\",\"0\",\"x\",\"x\",\"0\",\"x\",\"x\",\"1\",\"A\",\"5\",\"1\",\"A\",\"6\",\"1\",\"A\",\"7\",\"1\",\"0\",\"0\",\"0\",\"0\",\"0\",\"0\",\"0\",\"0\",\"PP\",\"0\",\"UP\"]"  sampletime=-1  sampletimestr=Inf  blockid=SPI2SPIMasterReadWrite
  SPI Master Read/Write1 : stm32f4_spi_lib/SPI Master Read//Write  configuration=Transaction  module=3  mode=Read/ Write  lastmodule=1  direction=Full-Duplex  dataformat=8bit/ FirstBit_MSB  prescaler=4  cpolcpha=CPOL_Low/ CPHA_1Edge  datacount=2  nssmode=Custom  nsspin=Not used  softnssport=E  softnsspin=0  sckpin=A5  misopin=A6  mosipin=A7  inputtypearray=[2 3 3]  outputtypearray=[3 7 3 3]  confstr="[\"SPI_Direction_2Lines_FullDuplex\",\"8b\",\"MSB\",\"Low\",\"1Edge\",\"4\",\"Soft\",\"0\",\"x\",\"x\",\"0\",\"x\",\"x\",\"1\",\"A\",\"5\",\"1\",\"A\",\"6\",\"1\",\"A\",\"7\",\"1\",\"0\",\"0\",\"0\",\"0\",\"0\",\"0\",\"0\",\"0\",\"PP\",\"0\",\"UP\"]"  sampletime=-1  sampletimestr=Inf  blockid=SPI2SPIMasterReadWrite1
  SPI Master Read/Write2 : stm32f4_spi_lib/SPI Master Read//Write  configuration=Transaction  module=3  mode=Read/ Write  lastmodule=1  direction=Full-Duplex  dataformat=8bit/ FirstBit_MSB  prescaler=4  cpolcpha=CPOL_Low/ CPHA_1Edge  datacount=2  nssmode=Custom  nsspin=Not used  softnssport=E  softnsspin=0  sckpin=A5  misopin=A6  mosipin=A7  inputtypearray=[2 3 3]  outputtypearray=[3 7 3 3]  confstr="[\"SPI_Direction_2Lines_FullDuplex\",\"8b\",\"MSB\",\"Low\",\"1Edge\",\"4\",\"Soft\",\"0\",\"x\",\"x\",\"0\",\"x\",\"x\",\"1\",\"A\",\"5\",\"1\",\"A\",\"6\",\"1\",\"A\",\"7\",\"1\",\"0\",\"0\",\"0\",\"0\",\"0\",\"0\",\"0\",\"0\",\"PP\",\"0\",\"UP\"]"  sampletime=-1  sampletimestr=Inf  blockid=SPI2SPIMasterReadWrite2
  Set regist 1 : Constant  Value=hex2dec('0')  OutDataTypeStr=uint8
  Set regist 2 : Constant  Value=hex2dec('0')  OutDataTypeStr=uint8
  Set register : Constant  Value=hex2dec('0')  OutDataTypeStr=uint8
  Take away sleepmode : Constant  Value=hex2dec('01')  OutDataTypeStr=uint8
  Take away sleepmode1 : Constant  Value=hex2dec('0')  OutDataTypeStr=uint8
  Take away sleepmode2 : Constant  Value=hex2dec('80')  OutDataTypeStr=uint8
  wires:
  SPI Master Read/Write/1 -> DUMMY1/1
  SPI Master Read/Write/2 -> DUMMY2/1
  SPI Master Read/Write/3 -> DUMMY3/1
  Bitwise Operator/1 -> SPI Master Read/Write/1
  Set regist 2/1 -> Bitwise Operator/2
  "PWR_MGMT_1 "/1 -> Bitwise Operator/1
  Take away sleepmode/1 -> SPI Master Read/Write/2
  SPI Master Read/Write1/1 -> DUMMY4/1
  SPI Master Read/Write1/2 -> DUMMY5/1
  SPI Master Read/Write1/3 -> DUMMY6/1
  Bitwise Operator1/1 -> SPI Master Read/Write1/1
  Set register/1 -> Bitwise Operator1/2
  PWR_MGMT_1 1/1 -> Bitwise Operator1/1
  Take away sleepmode1/1 -> SPI Master Read/Write1/2
  SPI Master Read/Write2/1 -> DUMMY7/1
  SPI Master Read/Write2/2 -> DUMMY8/1
  SPI Master Read/Write2/3 -> DUMMY9/1
  Bitwise Operator2/1 -> SPI Master Read/Write2/1
  Set regist 1/1 -> Bitwise Operator2/2
  PWR_MGMT_1 2/1 -> Bitwise Operator2/1
  Take away sleepmode2/1 -> SPI Master Read/Write2/2
